simulink model "s3"  (Simulink 7.4)
settings: Solver=ode45  StartTime=0.0  StopTime=10.0  RelTol=1e-3
libraries: dspsigops x1, dspsrcs4 x1, dspsnks4 x1
settings Model: Creator=ml43519  LastModifiedBy=ml43519

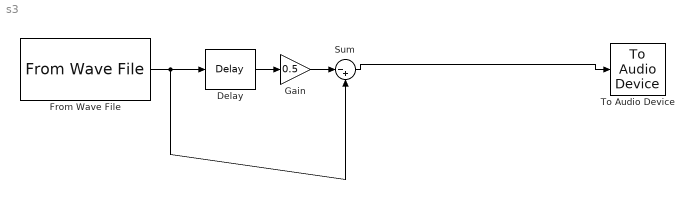
== system s3 ==
  Delay : dspsigops/Delay  dly_unit=Samples  delay=3000  ic_detail=off  dif_ic_for_ch=off  dif_ic_for_dly=off  ic=0  reset_popup=None
  From Wave File : dspsrcs4/From Wave File  FileName=0036434920_z332_a0.5_D3000.wav  SamplesPerFrame=1024  MinBufSize=1024  dType=double  bLoop=off  timesToPlay=1  restartMode=immediately after last sample  firstSampleOutput=off  lastSampleOutput=off
  Gain : Gain  Gain=0.5  ParameterDataType=fixdt(1, 16)  ParameterScaling=2^0  OutDataType=fixdt(1, 16)  OutScaling=2^0
  Sum : Sum  Inputs=|-+  OutDataType=fixdt(1, 16)  OutScaling=2^0
  To Audio Device : dspsnks4/To Audio Device  DialogController=dspDDGCreate  DialogControllerArgs=DataTag0  deviceName=Default  inheritSampleRate=on  sampleRate=44100  deviceDatatype=Determine from input data type  autoBufferSize=on  bufferSize=4096  queueDuration=1.0
  wires:
  Sum/1 -> To Audio Device/1
  Gain/1 -> Sum/1
  Delay/1 -> Gain/1
  From Wave File/1 -> Delay/1, Sum/2
